simulink model "fourteen_bus_partial_linear"  (R2020b)
settings: Solver=VariableStepAuto  StartTime=0.0  StopTime=1  RelTol=1e-3
libraries: powerlib x95, powerlib_meascontrol x2
(part 1 of 2)
settings Model: Creator=aayushyaagarwal  LastModifiedBy=aayushyaagarwal

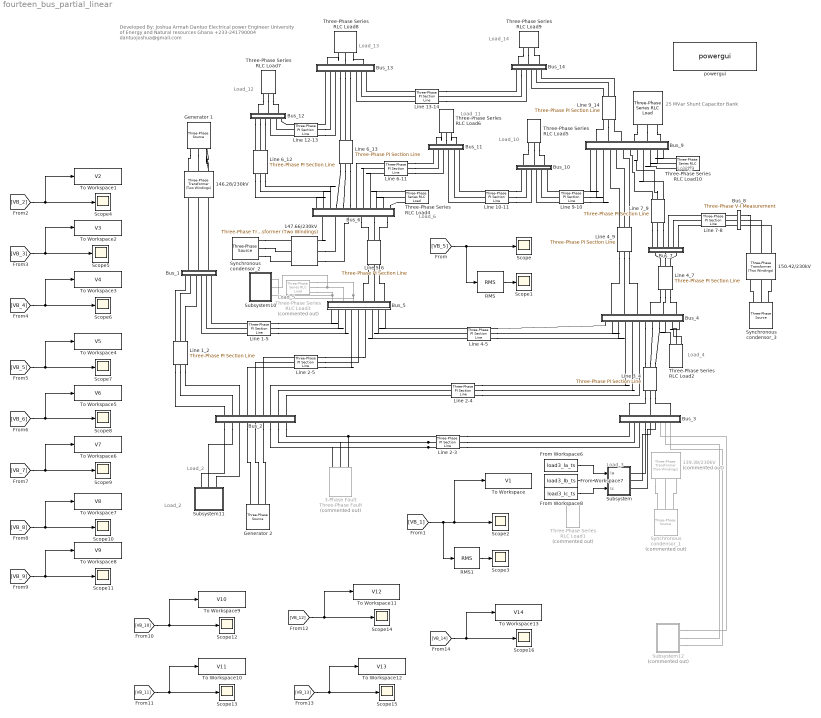
== system fourteen_bus_partial_linear ==
  note: Load_3
  note: Load_10
  note: Developed By:
      | Joshua Armah Dantuo
      | Electrical power Engineer
      | University of Energy and Natural resources
      | Ghana
      | +233-241790004
      | dantuojoshua@gmail.com
  note: Load_5
  note: Load_11
  note: Load_4
  note: Load_14
  note: Load_2
  note: Load_6
  note: Load_9
  note: Load_12
  note: Load_13
  note: 25 MVar Shunt
      | Capacitor Bank
  note: Load_2
  " " : powerlib/Elements/Three-Phase Series RLC Load  LConnTagsString=A|B|C  Configuration=Y (grounded)  NominalVoltage=230e3  Vabc=[1e3 1e3 1e3]  Vabcp=[1e3 1e3 1e3]  NominalFrequency=60  UnbalancedPower=off  ActivePower=0  InductivePower=0  CapacitivePower=25e6  Pabc=[10e3 9e3 11e3]  QLabc=[100 90 110]  QCabc=[100 90 110]  Pabcp=[10e3 9e3 11e3]  QLabcp=[100 90 110]  QCabcp=[100 90 110]  Measurements=None  LoadType=constant Z
  139.38/230kV : powerlib/Elements/Three-Phase Transformer (Two Windings)  Commented=on  Winding1Connection=Yg  Winding2Connection=Yg  CoreType=Three single-phase transformers  SetSaturation=off  Hysteresis=off  DataFile='hysteresis'  SetInitialFlux=off  Measurements=None  UNITS=pu  NominalPower=[ 120e6 , 60 ]  Winding1=[139.38e3 , 0.002 , 0.08 ]  Winding2=[ 230e3 , 0.002 , 0.08 ]  Rm=500  Lm=500  L0=0.5  Saturation=[ 0,0 ; 0.0024,1.2 ; 1.0,1.52 ]  InitialFluxes=[ 0.8 , -0.8 , 0.7 ]  BreakLoop=off  DiscreteSolver=Trapezoidal iterative  DataType=off  TransfoNumber=1
  146.28/230kV : powerlib/Elements/Three-Phase Transformer (Two Windings)  Winding1Connection=Yg  Winding2Connection=Yg  CoreType=Three single-phase transformers  SetSaturation=off  Hysteresis=off  DataFile='hysteresis'  SetInitialFlux=off  Measurements=None  UNITS=pu  NominalPower=[ 120e6 , 60 ]  Winding1=[146.28e3 , 0.002 , 0.08 ]  Winding2=[ 230e3 , 0.002 , 0.08 ]  Rm=500  Lm=500  L0=0.5  Saturation=[ 0,0 ; 0.0024,1.2 ; 1.0,1.52 ]  InitialFluxes=[ 0.8 , -0.8 , 0.7 ]  BreakLoop=off  DiscreteSolver=Trapezoidal iterative  DataType=off  TransfoNumber=1
  147.66/230kV : powerlib/Elements/Three-Phase Transformer (Two Windings)  Winding1Connection=Yg  Winding2Connection=Yg  CoreType=Three single-phase transformers  SetSaturation=off  Hysteresis=off  DataFile='hysteresis'  SetInitialFlux=off  Measurements=None  UNITS=pu  NominalPower=[ 120e6 , 60 ]  Winding1=[147.66e3 , 0.002 , 0.08 ]  Winding2=[ 230e3 , 0.002 , 0.08 ]  Rm=500  Lm=500  L0=0.5  Saturation=[ 0,0 ; 0.0024,1.2 ; 1.0,1.52 ]  InitialFluxes=[ 0.8 , -0.8 , 0.7 ]  BreakLoop=off  DiscreteSolver=Trapezoidal iterative  DataType=off  TransfoNumber=1
  150.42/230kV : powerlib/Elements/Three-Phase Transformer (Two Windings)  Winding1Connection=Yg  Winding2Connection=Yg  CoreType=Three single-phase transformers  SetSaturation=off  Hysteresis=off  DataFile='hysteresis'  SetInitialFlux=off  Measurements=None  UNITS=pu  NominalPower=[ 120e6 , 60 ]  Winding1=[150.42e3 , 0.002 , 0.08 ]  Winding2=[ 230e3 , 0.002 , 0.08 ]  Rm=500  Lm=500  L0=0.5  Saturation=[ 0,0 ; 0.0024,1.2 ; 1.0,1.52 ]  InitialFluxes=[ 0.8 , -0.8 , 0.7 ]  BreakLoop=off  DiscreteSolver=Trapezoidal iterative  DataType=off  TransfoNumber=1
  3-Phase Fault : powerlib/Elements/Three-Phase Fault  Commented=on  InitialStates=0  FaultA=on  FaultB=on  FaultC=on  GroundFault=on  SwitchTimes=[ 1 2]  External=off  SwitchStatus=NaN  FaultResistance=1e-3  GroundResistance=1e-3  SnubberResistance=inf  SnubberCapacitance=inf  Measurements=None
  Bus_1 : Subsystem
  Bus_10 : Subsystem
  Bus_11 : Subsystem
  Bus_12 : Subsystem
  Bus_13 : Subsystem
  Bus_14 : Subsystem
  Bus_2 : Subsystem
  Bus_3 : Subsystem
  Bus_4 : Subsystem
  Bus_5 : Subsystem
  Bus_6 : Subsystem
  Bus_7 : Subsystem
  Bus_8 : powerlib/Measurements/Three-Phase V-I Measurement  VoltageMeasurement=phase-to-phase  SetLabelV=on  LabelV=VB_8  Vpu=off  VpuLL=off  CurrentMeasurement=yes  SetLabelI=on  LabelI=IB_8  Ipu=off  Pbase=100e6  Vbase=500e3  OutputType=Complex  PhasorSimulation=off  PSBequivalent=0
  Bus_9 : Subsystem
  From Workspace6 : FromWorkspace  VariableName=load3_Ia_ts
  From Workspace7 : FromWorkspace  VariableName=load3_Ib_ts
  From Workspace8 : FromWorkspace  VariableName=load3_Ic_ts
  Generator 1 : powerlib/Electrical Sources/Three-Phase Source  InternalConnection=Yg  VoltagePhases=off  Voltage=(146280)*1.03071  PhaseAngle=3.7708  Voltage_phases=[25e3 25e3 25e3]/sqrt(3)  PhaseAngles_phases=[0 -120 +120]  Frequency=60  NonIdealSource=on  SpecifyImpedance=off  Resistance=0.8929  Inductance=16.58e-3  ShortCircuitLevel=100e6  BaseVoltage=146.28e3  XRratio=7  BusType=PV  Pref=163e6  Qref=0  Prefabc=[10e3, 10e3, 10e3]  Qrefabc=[0, 0, 0]  Qmin=-inf  Qmax=inf
  Generator 2 : powerlib/Electrical Sources/Three-Phase Source  InternalConnection=Yg  VoltagePhases=off  Voltage=(144210)*1.01655  PhaseAngle=-15.8323  Voltage_phases=[25e3 25e3 25e3]/sqrt(3)  PhaseAngles_phases=[0 -120 +120]  Frequency=60  NonIdealSource=on  SpecifyImpedance=off  Resistance=0.8929  Inductance=16.58e-3  ShortCircuitLevel=100e6  BaseVoltage=144.21e3  XRratio=7  BusType=PV  Pref=90e6  Qref=0  Prefabc=[10e3, 10e3, 10e3]  Qrefabc=[0, 0, 0]  Qmin=-inf  Qmax=inf
  Line 1-5 : powerlib/Elements/Three-Phase PI Section Line  LConnTagsString=a|b|c  RConnTagsString=A|B|C  Length=78.64  Frequency=60  Resistances=[ 0.3029 0.9086]  Inductances=[ 0.0033 0.0099]  Capacitances=[3.35e-7 1.01e-7]
  Line 10-11 : powerlib/Elements/Three-Phase PI Section Line  LConnTagsString=a|b|c  RConnTagsString=A|B|C  Length=4.93  Frequency=60  Resistances=[ 0.3667 1.1002]  Inductances=[ 0.0023 0.0068]  Capacitances=[1.22e-8 3.66e-8]
  Line 12-13 : powerlib/Elements/Three-Phase PI Section Line  LConnTagsString=a|b|c  RConnTagsString=A|B|C  Length=5.03  Frequency=60  Resistances=[ 0.9679 2.9038]  Inductances=[ 0.0023 0.0070]  Capacitances=[1.20e-8 3.59e-8]
  Line 13-14 : powerlib/Elements/Three-Phase PI Section Line  LConnTagsString=a|b|c  RConnTagsString=A|B|C  Length=6.64  Frequency=60  Resistances=[ 0.5676 1.7027]  Inductances=[ 0.0031 0.0092]  Capacitances=[9.06e-9 2.72e-9]
  Line 1_2 : powerlib/Elements/Three-Phase PI Section Line  LConnTagsString=a|b|c  RConnTagsString=A|B|C  Length=44.47  Frequency=60  Resistances=[ 0.1921 0.5763]  Inductances=[ 0.0016 0.0047]  Capacitances=[7.14e-9 2.14e-8]
  Line 2-3 : powerlib/Elements/Three-Phase PI Section Line  LConnTagsString=a|b|c  RConnTagsString=A|B|C  Length=68.47  Frequency=60  Resistances=[ 0.3026 0.9077]  Inductances=[ 0.0034 0.0101]  Capacitances=[3.29e-9 9.86e-8]
  Line 2-4 : powerlib/Elements/Three-Phase PI Section Line  LConnTagsString=a|b|c  RConnTagsString=A|B|C  Length=74.11  Frequency=60  Resistances=[ 0.3457 1.0370]  Inductances=[ 0.0028 0.0083]  Capacitances=[3.99e-9 1.20e-8]
  Line 2-5 : powerlib/Elements/Three-Phase PI Section Line  LConnTagsString=a|b|c  RConnTagsString=A|B|C  Length=61.18  Frequency=60  Resistances=[ 0.4104 1.2311]  Inductances=[ 0.0033 0.0100]  Capacitances=[3.34e-8 1.0e-8]
  Line 3_4 : powerlib/Elements/Three-Phase PI Section Line  LConnTagsString=a|b|c  RConnTagsString=A|B|C  Length=61.21  Frequency=60  Resistances=[ 0.4826 1.4479]  Inductances=[ 0.0033 0.0098]  Capacitances=[3.4e-9 1.02e-8]
  Line 4-5 : powerlib/Elements/Three-Phase PI Section Line  LConnTagsString=a|b|c  RConnTagsString=A|B|C  Length=18.47  Frequency=60  Resistances=[ 0.3186 0.9558]  Inductances=[ 0.0027 0.0080]  Capacitances=[4.17e-9 1.25e-8]
  Line 4_7 : powerlib/Elements/Three-Phase PI Section Line  LConnTagsString=a|b|c  RConnTagsString=A|B|C  Length=5.15  Frequency=60  Resistances=[ 0.0001 0.0003]  Inductances=[ 0.0475 0.1425]  Capacitances=[2.34e-10 7.02e-10]
  Line 4_9 : powerlib/Elements/Three-Phase PI Section Line  LConnTagsString=a|b|c  RConnTagsString=A|B|C  Length=8.39  Frequency=60  Resistances=[ 0.0001 0.0003]  Inductances=[ 0.0775 0.2325]  Capacitances=[1.43e-8 4.3e-8]
  Line 5_6 : powerlib/Elements/Three-Phase PI Section Line  LConnTagsString=a|b|c  RConnTagsString=A|B|C  Length=5.65  Frequency=60  Resistances=[ 0.0001 0.0003]  Inductances=[ 0.0522 0.1565]  Capacitances=[2.13e-10 6.39e-10]
  Line 6-11 : powerlib/Elements/Three-Phase PI Section Line  LConnTagsString=a|b|c  RConnTagsString=A|B|C  Length=5.02  Frequency=60  Resistances=[ 0.4172 1.2515]  Inductances=[ 0.0023 0.0070]  Capacitances=[1.20e-8 3.60e-8]
  Line 6_12 : powerlib/Elements/Three-Phase PI Section Line  LConnTagsString=a|b|c  RConnTagsString=A|B|C  Length=5.69  Frequency=60  Resistances=[ 0.4760 1.4281]  Inductances=[ 0.0026 0.0079]  Capacitances=[1.06e-8 3.17e-8]
  Line 6_13 : powerlib/Elements/Three-Phase PI Section Line  LConnTagsString=a|b|c  RConnTagsString=A|B|C  Length=4.06  Frequency=60  Resistances=[ 0.3590 1.0770]  Inductances=[ 0.0019 0.0056]  Capacitances=[1.48e-8 4.44e-8]
  Line 7-8 : powerlib/Elements/Three-Phase PI Section Line  LConnTagsString=a|b|c  RConnTagsString=A|B|C  Length=4.72  Frequency=60  Resistances=[ 0.0005 0.0014]  Inductances=[ 0.0022 0.0065]  Capacitances=[ 1.27e-8 3.82e-8]
  Line 7_9 : powerlib/Elements/Three-Phase PI Section Line  LConnTagsString=a|b|c  RConnTagsString=A|B|C  Length=3.73  Frequency=60  Resistances=[ 0.0006 0.0018]  Inductances=[ 0.0017 0.0052]  Capacitances=[ 1.61e-8 4.84e-8]
  Line 9-10 : powerlib/Elements/Three-Phase PI Section Line  LConnTagsString=a|b|c  RConnTagsString=A|B|C  Length=3.27  Frequency=60  Resistances=[ 0.2144 0.6431]  Inductances=[ 0.015 0.045]  Capacitances=[1.84e-9 5.52e-9]
  Line 9_14 : powerlib/Elements/Three-Phase PI Section Line  LConnTagsString=a|b|c  RConnTagsString=A|B|C  Length=69.85  Frequency=60  Resistances=[ 0.4788 1.4365]  Inductances=[ 0.027 0.081]  Capacitances=[1.03e-9 3.08e-9]
  RMS : powerlib_meascontrol/Measurements/RMS  TrueRMS=on  Freq=60  RMSInit=120  Ts=0
  RMS1 : powerlib_meascontrol/Measurements/RMS  TrueRMS=on  Freq=60  RMSInit=120  Ts=0
  Scope{,1..16} (17 alike) : Scope
  Subsystem : Subsystem
  Subsystem10 : Subsystem
  Subsystem11 : Subsystem
  Subsystem12 : Subsystem  Commented=on
  Synchronous condensor_1 : powerlib/Electrical Sources/Three-Phase Source  Commented=on  InternalConnection=Yg  VoltagePhases=off  Voltage=(139380)*1.01137  PhaseAngle=-34.48  Voltage_phases=[25e3 25e3 25e3]/sqrt(3)  PhaseAngles_phases=[0 -120 +120]  Frequency=60  NonIdealSource=on  SpecifyImpedance=off  Resistance=0.8929  Inductance=16.58e-3  ShortCircuitLevel=100e6  BaseVoltage=139.38e3  XRratio=7  BusType=PV  Pref=0  Qref=50.096e6  Prefabc=[10e3, 10e3, 10e3]  Qrefabc=[0, 0, 0]  Qmin=-inf  Qmax=inf
  Synchronous condensor_2 : powerlib/Electrical Sources/Three-Phase Source  InternalConnection=Yg  VoltagePhases=off  Voltage=(147660)*0.984306  PhaseAngle=-36.2022  Voltage_phases=[25e3 25e3 25e3]/sqrt(3)  PhaseAngles_phases=[0 -120 +120]  Frequency=60  NonIdealSource=on  SpecifyImpedance=off  Resistance=0.8929  Inductance=16.58e-3  ShortCircuitLevel=100e6  BaseVoltage=147.66e3  XRratio=7  BusType=PQ  Pref=0  Qref=25.276e6  Prefabc=[10e3, 10e3, 10e3]  Qrefabc=[0, 0, 0]  Qmin=-inf  Qmax=inf
  Synchronous condensor_3 : powerlib/Electrical Sources/Three-Phase Source  InternalConnection=Yg  VoltagePhases=off  Voltage=(150420)*0.995122  PhaseAngle=-36.1424  Voltage_phases=[25e3 25e3 25e3]/sqrt(3)  PhaseAngles_phases=[0 -120 +120]  Frequency=60  NonIdealSource=on  SpecifyImpedance=off  Resistance=0.8929  Inductance=16.58e-3  ShortCircuitLevel=100e6  BaseVoltage=150.42e3  XRratio=7  BusType=PQ  Pref=0  Qref=30.144e6  Prefabc=[10e3, 10e3, 10e3]  Qrefabc=[0, 0, 0]  Qmin=-inf  Qmax=inf
  Three-Phase Series RLC Load1 : powerlib/Elements/Three-Phase Series RLC Load  Commented=on  LConnTagsString=A|B|C  Configuration=Y (grounded)  NominalVoltage=(230000)*0.92821  Vabc=[1e3 1e3 1e3]  Vabcp=[1e3 1e3 1e3]  NominalFrequency=60  UnbalancedPower=off  ActivePower=113.04e6  InductivePower=22.8e6  CapacitivePower=0  Pabc=[10e3 9e3 11e3]  QLabc=[100 90 110]  QCabc=[100 90 110]  Pabcp=[10e3 9e3 11e3]  QLabcp=[100 90 110]  QCabcp=[100 90 110]  Measurements=None  LoadType=constant PQ
  Three-Phase Series RLC Load10 : powerlib/Elements/Three-Phase Series RLC Load  LConnTagsString=A|B|C  Configuration=Y (grounded)  NominalVoltage=(230000)*0.942986  Vabc=[1e3 1e3 1e3]  Vabcp=[1e3 1e3 1e3]  NominalFrequency=60  UnbalancedPower=off  ActivePower=35.4e6  InductivePower=19.92e6  CapacitivePower=0  Pabc=[10e3 9e3 11e3]  QLabc=[100 90 110]  QCabc=[100 90 110]  Pabcp=[10e3 9e3 11e3]  QLabcp=[100 90 110]  QCabcp=[100 90 110]  Measurements=None  LoadType=constant PQ
  Three-Phase Series RLC Load2 : powerlib/Elements/Three-Phase Series RLC Load  LConnTagsString=A|B|C  Configuration=Y (grounded)  NominalVoltage=(230000)*0.927953  Vabc=[1e3 1e3 1e3]  Vabcp=[1e3 1e3 1e3]  NominalFrequency=60  UnbalancedPower=off  ActivePower=57.36e6  InductivePower=0  CapacitivePower=4.68e6  Pabc=[10e3 9e3 11e3]  QLabc=[100 90 110]  QCabc=[100 90 110]  Pabcp=[10e3 9e3 11e3]  QLabcp=[100 90 110]  QCabcp=[100 90 110]  Measurements=None  LoadType=constant PQ
  Three-Phase Series RLC Load3 : powerlib/Elements/Three-Phase Series RLC Load  Commented=on  LConnTagsString=A|B|C  Configuration=Y (grounded)  NominalVoltage=(230000)*0.931217  Vabc=[1e3 1e3 1e3]  Vabcp=[1e3 1e3 1e3]  NominalFrequency=60  UnbalancedPower=off  ActivePower=9.12e6  InductivePower=1.92e6  CapacitivePower=0  Pabc=[10e3 9e3 11e3]  QLabc=[100 90 110]  QCabc=[100 90 110]  Pabcp=[10e3 9e3 11e3]  QLabcp=[100 90 110]  QCabcp=[100 90 110]  Measurements=None  LoadType=constant PQ
  Three-Phase Series RLC Load4 : powerlib/Elements/Three-Phase Series RLC Load  LConnTagsString=A|B|C  Configuration=Y (grounded)  NominalVoltage=(230000)*0.942548  Vabc=[1e3 1e3 1e3]  Vabcp=[1e3 1e3 1e3]  NominalFrequency=60  UnbalancedPower=off  ActivePower=13.44e6  InductivePower=9e6  CapacitivePower=0  Pabc=[10e3 9e3 11e3]  QLabc=[100 90 110]  QCabc=[100 90 110]  Pabcp=[10e3 9e3 11e3]  QLabcp=[100 90 110]  QCabcp=[100 90 110]  Measurements=None  LoadType=constant PQ
  Three-Phase Series RLC Load5 : powerlib/Elements/Three-Phase Series RLC Load  LConnTagsString=A|B|C  Configuration=Y (grounded)  NominalVoltage=(230000)*0.942502  Vabc=[1e3 1e3 1e3]  Vabcp=[1e3 1e3 1e3]  NominalFrequency=60  UnbalancedPower=off  ActivePower=10.8e6  InductivePower=6.96e6  CapacitivePower=0  Pabc=[10e3 9e3 11e3]  QLabc=[100 90 110]  QCabc=[100 90 110]  Pabcp=[10e3 9e3 11e3]  QLabcp=[100 90 110]  QCabcp=[100 90 110]  Measurements=None  LoadType=constant PQ
  Three-Phase Series RLC Load6 : powerlib/Elements/Three-Phase Series RLC Load  LConnTagsString=A|B|C  Configuration=Y (grounded)  NominalVoltage=(230000)*0.942338  Vabc=[1e3 1e3 1e3]  Vabcp=[1e3 1e3 1e3]  NominalFrequency=60  UnbalancedPower=off  ActivePower=4.2e6  InductivePower=2.16e6  CapacitivePower=0  Pabc=[10e3 9e3 11e3]  QLabc=[100 90 110]  QCabc=[100 90 110]  Pabcp=[10e3 9e3 11e3]  QLabcp=[100 90 110]  QCabcp=[100 90 110]  Measurements=None  LoadType=constant PQ
  Three-Phase Series RLC Load7 : powerlib/Elements/Three-Phase Series RLC Load  LConnTagsString=A|B|C  Configuration=Y (grounded)  NominalVoltage=(230000)*0.941818  Vabc=[1e3 1e3 1e3]  Vabcp=[1e3 1e3 1e3]  NominalFrequency=60  UnbalancedPower=off  ActivePower=7.32e6  InductivePower=1.92e6  CapacitivePower=0  Pabc=[10e3 9e3 11e3]  QLabc=[100 90 110]  QCabc=[100 90 110]  Pabcp=[10e3 9e3 11e3]  QLabcp=[100 90 110]  QCabcp=[100 90 110]  Measurements=None  LoadType=constant PQ
  Three-Phase Series RLC Load8 : powerlib/Elements/Three-Phase Series RLC Load  LConnTagsString=A|B|C  Configuration=Y (grounded)  NominalVoltage=(230000)*0.941642  Vabc=[1e3 1e3 1e3]  Vabcp=[1e3 1e3 1e3]  NominalFrequency=60  UnbalancedPower=off  ActivePower=16.2e6  InductivePower=6.96e6  CapacitivePower=0  Pabc=[10e3 9e3 11e3]  QLabc=[100 90 110]  QCabc=[100 90 110]  Pabcp=[10e3 9e3 11e3]  QLabcp=[100 90 110]  QCabcp=[100 90 110]  Measurements=None  LoadType=constant PQ
  Three-Phase Series RLC Load9 : powerlib/Elements/Three-Phase Series RLC Load  LConnTagsString=A|B|C  Configuration=Y (grounded)  NominalVoltage=(230000)*0.941422  Vabc=[1e3 1e3 1e3]  Vabcp=[1e3 1e3 1e3]  NominalFrequency=60  UnbalancedPower=off  ActivePower=17.88e6  InductivePower=6e6  CapacitivePower=0  Pabc=[10e3 9e3 11e3]  QLabc=[100 90 110]  QCabc=[100 90 110]  Pabcp=[10e3 9e3 11e3]  QLabcp=[100 90 110]  QCabcp=[100 90 110]  Measurements=None  LoadType=constant PQ
  To Workspace : ToWorkspace  VariableName=V1  SaveFormat=Timeseries  SampleTime=-1
  To Workspace1 : ToWorkspace  VariableName=V2  SaveFormat=Timeseries  SampleTime=-1
  To Workspace10 : ToWorkspace  VariableName=V11  SaveFormat=Timeseries  SampleTime=-1
  To Workspace11 : ToWorkspace  VariableName=V12  SaveFormat=Timeseries  SampleTime=-1
  To Workspace12 : ToWorkspace  VariableName=V13  SaveFormat=Timeseries  SampleTime=-1
  To Workspace13 : ToWorkspace  VariableName=V14  SaveFormat=Timeseries  SampleTime=-1
  To Workspace2 : ToWorkspace  VariableName=V3  SaveFormat=Timeseries  SampleTime=-1
  To Workspace3 : ToWorkspace  VariableName=V4  SaveFormat=Timeseries  SampleTime=-1
  To Workspace4 : ToWorkspace  VariableName=V5  SaveFormat=Timeseries  SampleTime=-1
  To Workspace5 : ToWorkspace  VariableName=V6  SaveFormat=Timeseries  SampleTime=-1
  To Workspace6 : ToWorkspace  VariableName=V7  SaveFormat=Timeseries  SampleTime=-1
  To Workspace7 : ToWorkspace  VariableName=V8  SaveFormat=Timeseries  SampleTime=-1
  To Workspace8 : ToWorkspace  VariableName=V9  SaveFormat=Timeseries  SampleTime=-1
  To Workspace9 : ToWorkspace  VariableName=V10  SaveFormat=Timeseries  SampleTime=-1
  powergui : powerlib/powergui  Priority=1  SimulationMode=Discrete  SampleTime=50e-6  frequency=60  Iterations=50  frequencyindice=60  Pbase=120e6  ErrMax=0.0001  UnitsV=kV  UnitsW=MW  buscounter=0  FunctionMessages=off  echomessages=off  EnableUseOfTLC=off  CurrentSourceSwitches=off  DisableSnubberDevices=off  DisableRonSwitches=off  DisableVfSwitches=off  DisplayEquations=off  AutomaticDiscreteSolvers=off  SolverType=Tustin/Backward Euler (TBE)  Interpol=off  ExternalGateDelay=off  methode=off  Ts=100  x0status=steady  SPID=on  SwTol=0  HookPort=off  NonlinearTolerance=1e-4  nMaxIteration=100  ContinueOnMaxIteration=off  RestoreLinks=warning  ResistiveCurrentMeasurement=off  Frange=[0:2:500]  Ylog=off  Xlog=on  ShowGrid=off  save=off  variable=ZData  structure=0  ZoomFFT=off  StartTime=0.0  cycles=1  DisplayStyle=1  fundamental=60  FreqAxis=off  MaxFrequency=1000  frequencyindicesteady=1  RmsSteady=1  display=off
  wires:
  [VB_4] -> To Workspace3/1, Scope6/1
  [VB_8] -> To Workspace7/1, Scope10/1
  RMS1/1 -> Scope3/1
  [VB_2] -> To Workspace1/1, Scope4/1
  [VB_7] -> To Workspace6/1, Scope9/1
  [VB_12] -> To Workspace11/1, Scope14/1
  [VB_13] -> To Workspace12/1, Scope15/1
  RMS/1 -> Scope1/1
  [VB_10] -> To Workspace9/1, Scope12/1
  [VB_5] -> RMS/1, Scope/1
  [VB_6] -> To Workspace5/1, Scope8/1
  [VB_14] -> To Workspace13/1, Scope16/1
  [VB_11] -> To Workspace10/1, Scope13/1
  [VB_1] -> RMS1/1, To Workspace/1, Scope2/1
  [VB_5] -> To Workspace4/1, Scope7/1
  [VB_3] -> To Workspace2/1, Scope5/1
  [VB_9] -> To Workspace8/1, Scope11/1
  From Workspace6/1 -> Subsystem/1(Ia)
  From Workspace7/1 -> Subsystem/2(Ib)
  From Workspace8/1 -> Subsystem/3(Ic)
  connections:
  Bus_2/RConn9 -- 3-Phase Fault/LConn3 -- Line 2-3/LConn1
  Line 2-3/LConn3 -- Bus_2/RConn7 -- 3-Phase Fault/LConn1
  Line 2-3/LConn2 -- Bus_2/RConn8 -- 3-Phase Fault/LConn2
  Line 7_9/RConn1 -- Bus_7/RConn1
  Bus_2/RConn6 -- Generator 2/RConn3
  Line 5_6/RConn1 -- Bus_5/LConn4
  Bus_8/LConn1 -- Line 7-8/RConn1
  Line 12-13/LConn1 -- Bus_12/RConn6
  Three-Phase Series RLC Load4/LConn2 -- Bus_6/RConn11
  Line 6-11/RConn3 -- Bus_11/RConn3
  Line 6-11/RConn2 -- Bus_11/RConn2
  Line 1_2/RConn1 -- Bus_2/LConn1
  Line 6_12/RConn3 -- Bus_6/RConn3
  Line 5_6/RConn2 -- Bus_5/LConn5
  Line 10-11/LConn1 -- Bus_11/RConn6
  Line 1-5/RConn3 -- Bus_5/RConn3
  Line 10-11/RConn3 -- Bus_10/RConn3
  Three-Phase Series RLC Load8/LConn1 -- Bus_13/LConn1
  Line 12-13/LConn2 -- Bus_12/RConn5
  Line 2-4/RConn3 -- Bus_4/RConn6
  Line 2-4/LConn2 -- Bus_2/LConn8
  Three-Phase Series RLC Load10/LConn2 -- Bus_9/RConn11
  Synchronous condensor_3/RConn3 -- 150.42/230kV/LConn3
  Bus_2/RConn4 -- Generator 2/RConn1
  Three-Phase Series RLC Load3/LConn3 -- Subsystem10/RConn3 -- Bus_5/LConn1
  Synchronous condensor_2/RConn3 -- 147.66/230kV/LConn3
  Three-Phase Series RLC Load7/LConn2 -- Bus_12/LConn2
  Line 2-3/RConn1 -- Bus_3/RConn1
  Line 6_13/RConn3 -- Bus_6/RConn6
  " "/LConn2 -- Bus_9/LConn5
  Line 13-14/LConn3 -- Bus_13/RConn7
  Synchronous condensor_1/RConn3 -- 139.38/230kV/LConn3
  Bus_9/LConn3 -- Line 9_14/RConn3
  Three-Phase Series RLC Load9/LConn2 -- Bus_14/LConn2
  Bus_12/RConn3 -- Line 6_12/LConn3
  Line 4-5/RConn2 -- Bus_4/RConn2
  Line 4_9/LConn1 -- Bus_9/RConn4
  Line 4-5/RConn1 -- Bus_4/RConn1
  Line 6_12/RConn2 -- Bus_6/RConn2
  Line 2-5/LConn3 -- Bus_2/LConn4
  Line 4_7/RConn2 -- Bus_4/LConn5
  147.66/230kV/RConn2 -- Bus_6/LConn2
  139.38/230kV/LConn1 -- Synchronous condensor_1/RConn1
  Line 6_13/RConn2 -- Bus_6/RConn5
  Line 9-10/RConn1 -- Bus_9/RConn1
  Line 12-13/RConn1 -- Bus_13/RConn1
  Line 4_9/LConn2 -- Bus_9/RConn5
  Three-Phase Series RLC Load9/LConn1 -- Bus_14/LConn1
  Three-Phase Series RLC Load5/LConn1 -- Bus_10/LConn1
  Line 1-5/LConn2 -- Bus_1/RConn5
  Line 3_4/RConn2 -- Bus_3/LConn2
  Line 2-4/LConn1 -- Bus_2/LConn7
  Bus_6/LConn5 -- Line 5_6/LConn2
  Line 3_4/RConn3 -- Bus_3/LConn3
  Three-Phase Series RLC Load5/LConn3 -- Bus_10/LConn3
  Line 4_9/LConn3 -- Bus_9/RConn6
  Synchronous condensor_3/RConn1 -- 150.42/230kV/LConn1
  Three-Phase Series RLC Load3/LConn1 -- Subsystem10/RConn1 -- Bus_5/LConn3
  Three-Phase Series RLC Load8/LConn3 -- Bus_13/LConn3
  Line 2-3/RConn2 -- Bus_3/RConn2
  " "/LConn1 -- Bus_9/LConn4
  Line 9-10/RConn2 -- Bus_9/RConn2
  Bus_12/RConn1 -- Line 6_12/LConn1
  Line 6-11/RConn1 -- Bus_11/RConn1
  Line 12-13/LConn3 -- Bus_12/RConn4
  Three-Phase Series RLC Load4/LConn3 -- Bus_6/RConn12
  Line 1_2/RConn3 -- Bus_2/LConn3
  Line 1-5/LConn3 -- Bus_1/RConn4
  Line 2-5/RConn2 -- Bus_5/RConn5
  150.42/230kV/RConn2 -- Bus_8/RConn2
  Synchronous condensor_3/RConn2 -- 150.42/230kV/LConn2
  147.66/230kV/RConn3 -- Bus_6/LConn3
  Line 7_9/LConn1 -- Bus_9/RConn7
  Line 1-5/LConn1 -- Bus_1/RConn6
  Line 1_2/RConn2 -- Bus_2/LConn2
  Bus_14/RConn2 -- Line 13-14/RConn2
  Line 5_6/RConn3 -- Bus_5/LConn6
  Line 6_13/RConn1 -- Bus_6/RConn4
  Bus_13/RConn6 -- Line 6_13/LConn3
  Line 4_7/LConn1 -- Bus_7/LConn1
  Three-Phase Series RLC Load6/LConn1 -- Bus_11/LConn1
  Generator 1/RConn2 -- 146.28/230kV/LConn2
  Line 4-5/LConn3 -- Bus_5/RConn7
  Line 6-11/LConn1 -- Bus_6/RConn7
  Three-Phase Series RLC Load9/LConn3 -- Bus_14/LConn3
  Line 6_12/RConn1 -- Bus_6/RConn1
  Bus_4/RConn8 -- Line 3_4/LConn2
  Bus_8/LConn3 -- Line 7-8/RConn3
  Three-Phase Series RLC Load7/LConn3 -- Bus_12/LConn3
  Line 2-3/RConn3 -- Bus_3/RConn3
  Line 6-11/LConn2 -- Bus_6/RConn8
  Line 6-11/LConn3 -- Bus_6/RConn9
  Three-Phase Series RLC Load2/LConn2 -- Bus_4/RConn11
  Three-Phase Series RLC Load4/LConn1 -- Bus_6/RConn10
  Line 4-5/LConn1 -- Bus_5/RConn9
  Bus_6/LConn4 -- Line 5_6/LConn1
  Line 2-5/RConn3 -- Bus_5/RConn4
  Line 1-5/RConn1 -- Bus_5/RConn1
  Line 3_4/RConn1 -- Bus_3/LConn1
  Line 7-8/LConn3 -- Bus_7/RConn6
  Bus_8/RConn1 -- 150.42/230kV/RConn1
  Line 7_9/RConn2 -- Bus_7/RConn2
  Line 1-5/RConn2 -- Bus_5/RConn2
  Line 10-11/RConn1 -- Bus_10/RConn1
  Line 7-8/LConn1 -- Bus_7/RConn4
  Line 13-14/RConn3 -- Bus_14/RConn3
  Bus_4/RConn7 -- Line 3_4/LConn1
  Line 9_14/LConn1 -- Bus_14/RConn4
  Line 10-11/LConn2 -- Bus_11/RConn5
  Synchronous condensor_2/RConn1 -- 147.66/230kV/LConn1
  Line 4_9/RConn2 -- Bus_4/LConn2
  Line 9_14/RConn2 -- Bus_9/LConn2
  Line 2-4/RConn2 -- Bus_4/RConn5
  Line 9-10/LConn3 -- Bus_10/RConn4
  Line 9-10/LConn1 -- Bus_10/RConn6
  Synchronous condensor_1/RConn2 -- 139.38/230kV/LConn2
  Line 9-10/RConn3 -- Bus_9/RConn3
  Three-Phase Series RLC Load2/LConn3 -- Bus_4/RConn12
  Line 9-10/LConn2 -- Bus_10/RConn5
  Bus_12/RConn2 -- Line 6_12/LConn2
  Line 4-5/LConn2 -- Bus_5/RConn8
  Line 1_2/LConn3 -- Bus_1/RConn3
  Line 4_7/RConn1 -- Bus_4/LConn4
  Bus_2/LConn5 -- Line 2-5/LConn2
  Line 4-5/RConn3 -- Bus_4/RConn3
  " "/LConn3 -- Bus_9/LConn6
  Line 10-11/LConn3 -- Bus_11/RConn4
  Bus_13/RConn5 -- Line 6_13/LConn2
  Three-Phase Series RLC Load10/LConn1 -- Bus_9/RConn12
  Line 7_9/LConn3 -- Bus_9/RConn9
  Synchronous condensor_2/RConn2 -- 147.66/230kV/LConn2
  Line 13-14/LConn2 -- Bus_13/RConn8
  146.28/230kV/LConn1 -- Generator 1/RConn1
  Bus_4/RConn9 -- Line 3_4/LConn3
  Line 4_7/LConn3 -- Bus_7/LConn3
  Line 12-13/RConn3 -- Bus_13/RConn3
  Bus_8/LConn2 -- Line 7-8/RConn2
  Line 9_14/LConn2 -- Bus_14/RConn5
  Bus_9/LConn1 -- Line 9_14/RConn1
  Line 1_2/LConn1 -- Bus_1/RConn1
  Line 7-8/LConn2 -- Bus_7/RConn5
  Line 13-14/RConn1 -- Bus_14/RConn1
  Line 1_2/LConn2 -- Bus_1/RConn2
  Line 10-11/RConn2 -- Bus_10/RConn2
  150.42/230kV/RConn3 -- Bus_8/RConn3
  Line 4_7/RConn3 -- Bus_4/LConn6
  Line 4_9/RConn3 -- Bus_4/LConn3
  Three-Phase Series RLC Load7/LConn1 -- Bus_12/LConn1
  Three-Phase Series RLC Load10/LConn3 -- Bus_9/RConn10
  Line 7_9/RConn3 -- Bus_7/RConn3
  Bus_6/LConn6 -- Line 5_6/LConn3
  Bus_7/LConn2 -- Line 4_7/LConn2
  Line 2-5/RConn1 -- Bus_5/RConn6
  Three-Phase Series RLC Load6/LConn3 -- Bus_11/LConn3
  Line 2-5/LConn1 -- Bus_2/LConn6
  Line 4_9/RConn1 -- Bus_4/LConn1
  Line 9_14/LConn3 -- Bus_14/RConn6
  Three-Phase Series RLC Load5/LConn2 -- Bus_10/LConn2
  Line 7_9/LConn2 -- Bus_9/RConn8
  Line 2-4/LConn3 -- Bus_2/LConn9
  Three-Phase Series RLC Load3/LConn2 -- Subsystem10/RConn2 -- Bus_5/LConn2
  Line 13-14/LConn1 -- Bus_13/RConn9
  147.66/230kV/RConn1 -- Bus_6/LConn1
  Line 2-4/RConn1 -- Bus_4/RConn4
  Line 12-13/RConn2 -- Bus_13/RConn2
  Three-Phase Series RLC Load2/LConn1 -- Bus_4/RConn10
  Bus_2/RConn5 -- Generator 2/RConn2
  Generator 1/RConn3 -- 146.28/230kV/LConn3
  Three-Phase Series RLC Load8/LConn2 -- Bus_13/LConn2
  Three-Phase Series RLC Load6/LConn2 -- Bus_11/LConn2
  Bus_13/RConn4 -- Line 6_13/LConn1
  Bus_1/LConn2 -- 146.28/230kV/RConn2
  Bus_1/LConn3 -- 146.28/230kV/RConn1
  Bus_1/LConn1 -- 146.28/230kV/RConn3
  Bus_2/RConn2 -- Subsystem11/RConn2
  Bus_2/RConn1 -- Subsystem11/RConn1
  Subsystem11/RConn3 -- Bus_2/RConn3
  Bus_3/RConn4 -- Subsystem/RConn1
  Bus_3/RConn5 -- Subsystem/RConn2
  Bus_3/RConn6 -- Subsystem/RConn3
  Subsystem12/RConn1 -- Bus_3/RConn7
  Subsystem12/RConn2 -- Bus_3/RConn8
  Subsystem12/RConn3 -- Bus_3/RConn9

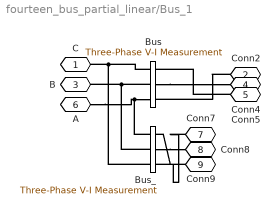
== system fourteen_bus_partial_linear/Bus_1 ==
  Bus : powerlib/Measurements/Three-Phase V-I Measurement  VoltageMeasurement=phase-to-phase  SetLabelV=on  LabelV=VB_1  Vpu=off  VpuLL=off  CurrentMeasurement=yes  SetLabelI=on  LabelI=IB_1  Ipu=off  Pbase=100e6  Vbase=500e3  OutputType=Complex  PhasorSimulation=off  PSBequivalent=0
  Bus_ : powerlib/Measurements/Three-Phase V-I Measurement  VoltageMeasurement=phase-to-phase  SetLabelV=on  LabelV=V_B1  Vpu=off  VpuLL=off  CurrentMeasurement=yes  SetLabelI=on  LabelI=I_B1  Ipu=off  Pbase=100e6  Vbase=500e3  OutputType=Complex  PhasorSimulation=off  PSBequivalent=0
  C : PMIOPort  Side=Left
  Conn2 : PMIOPort  Port=2  Side=Right
  B : PMIOPort  Port=3  Side=Left
  Conn4 : PMIOPort  Port=4  Side=Right
  Conn5 : PMIOPort  Port=5  Side=Right
  A : PMIOPort  Port=6  Side=Left
  Conn7 : PMIOPort  Port=7  Side=Right
  Conn8 : PMIOPort  Port=8  Side=Right
  Conn9 : PMIOPort  Port=9  Side=Right
  connections:
  A/RConn1 -- Bus_/LConn1 -- Bus/LConn3
  Bus/RConn2 -- Conn4/RConn1
  Bus_/RConn2 -- Conn8/RConn1
  Bus/LConn2 -- Bus_/LConn2 -- B/RConn1
  Bus/LConn1 -- Bus_/LConn3 -- C/RConn1
  Conn5/RConn1 -- Bus/RConn1
  Conn2/RConn1 -- Bus/RConn3
  Conn9/RConn1 -- Bus_/RConn1
  Conn7/RConn1 -- Bus_/RConn3

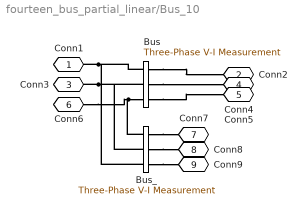
== system fourteen_bus_partial_linear/Bus_10 ==
  Bus : powerlib/Measurements/Three-Phase V-I Measurement  VoltageMeasurement=phase-to-phase  SetLabelV=on  LabelV=VB_10  Vpu=off  VpuLL=off  CurrentMeasurement=yes  SetLabelI=on  LabelI=IB_10  Ipu=off  Pbase=100e6  Vbase=500e3  OutputType=Complex  PhasorSimulation=off  PSBequivalent=0
  Bus_ : powerlib/Measurements/Three-Phase V-I Measurement  VoltageMeasurement=phase-to-phase  SetLabelV=on  LabelV=V_B10  Vpu=off  VpuLL=off  CurrentMeasurement=yes  SetLabelI=on  LabelI=I_B10  Ipu=off  Pbase=100e6  Vbase=500e3  OutputType=Complex  PhasorSimulation=off  PSBequivalent=0
  Conn1 : PMIOPort  Side=Left
  Conn2 : PMIOPort  Port=2  Side=Right
  Conn3 : PMIOPort  Port=3  Side=Left
  Conn4 : PMIOPort  Port=4  Side=Right
  Conn5 : PMIOPort  Port=5  Side=Right
  Conn6 : PMIOPort  Port=6  Side=Left
  Conn7 : PMIOPort  Port=7  Side=Right
  Conn8 : PMIOPort  Port=8  Side=Right
  Conn9 : PMIOPort  Port=9  Side=Right
  connections:
  Conn1/RConn1 -- Bus_/LConn3 -- Bus/LConn1
  Conn3/RConn1 -- Bus_/LConn2 -- Bus/LConn2
  Bus_/RConn2 -- Conn8/RConn1
  Bus/RConn2 -- Conn4/RConn1
  Bus/LConn3 -- Bus_/LConn1 -- Conn6/RConn1
  Bus_/RConn1 -- Conn7/RConn1
  Bus_/RConn3 -- Conn9/RConn1
  Bus/RConn1 -- Conn2/RConn1
  Bus/RConn3 -- Conn5/RConn1

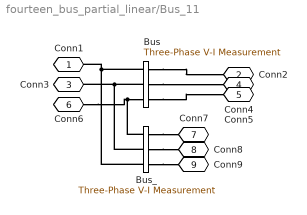
== system fourteen_bus_partial_linear/Bus_11 ==
  Bus : powerlib/Measurements/Three-Phase V-I Measurement  VoltageMeasurement=phase-to-phase  SetLabelV=on  LabelV=VB_11  Vpu=off  VpuLL=off  CurrentMeasurement=yes  SetLabelI=on  LabelI=IB_11  Ipu=off  Pbase=100e6  Vbase=500e3  OutputType=Complex  PhasorSimulation=off  PSBequivalent=0
  Bus_ : powerlib/Measurements/Three-Phase V-I Measurement  VoltageMeasurement=phase-to-phase  SetLabelV=on  LabelV=V_B11  Vpu=off  VpuLL=off  CurrentMeasurement=yes  SetLabelI=on  LabelI=I_B11  Ipu=off  Pbase=100e6  Vbase=500e3  OutputType=Complex  PhasorSimulation=off  PSBequivalent=0
  Conn1 : PMIOPort  Side=Left
  Conn2 : PMIOPort  Port=2  Side=Right
  Conn3 : PMIOPort  Port=3  Side=Left
  Conn4 : PMIOPort  Port=4  Side=Right
  Conn5 : PMIOPort  Port=5  Side=Right
  Conn6 : PMIOPort  Port=6  Side=Left
  Conn7 : PMIOPort  Port=7  Side=Right
  Conn8 : PMIOPort  Port=8  Side=Right
  Conn9 : PMIOPort  Port=9  Side=Right
  connections:
  Bus/RConn3 -- Conn5/RConn1
  Bus/RConn1 -- Conn2/RConn1
  Bus_/RConn3 -- Conn9/RConn1
  Bus_/RConn1 -- Conn7/RConn1
  Conn6/RConn1 -- Bus_/LConn1 -- Bus/LConn3
  Bus/RConn2 -- Conn4/RConn1
  Bus_/RConn2 -- Conn8/RConn1
  Bus/LConn2 -- Bus_/LConn2 -- Conn3/RConn1
  Bus/LConn1 -- Conn1/RConn1 -- Bus_/LConn3

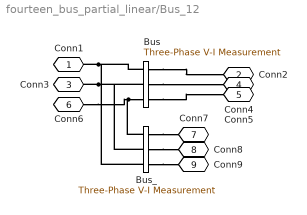
== system fourteen_bus_partial_linear/Bus_12 ==
  Bus : powerlib/Measurements/Three-Phase V-I Measurement  VoltageMeasurement=phase-to-phase  SetLabelV=on  LabelV=VB_12  Vpu=off  VpuLL=off  CurrentMeasurement=yes  SetLabelI=on  LabelI=IB_12  Ipu=off  Pbase=100e6  Vbase=500e3  OutputType=Complex  PhasorSimulation=off  PSBequivalent=0
  Bus_ : powerlib/Measurements/Three-Phase V-I Measurement  VoltageMeasurement=phase-to-phase  SetLabelV=on  LabelV=V_B12  Vpu=off  VpuLL=off  CurrentMeasurement=yes  SetLabelI=on  LabelI=I_B12  Ipu=off  Pbase=100e6  Vbase=500e3  OutputType=Complex  PhasorSimulation=off  PSBequivalent=0
  Conn1 : PMIOPort  Side=Left
  Conn2 : PMIOPort  Port=2  Side=Right
  Conn3 : PMIOPort  Port=3  Side=Left
  Conn4 : PMIOPort  Port=4  Side=Right
  Conn5 : PMIOPort  Port=5  Side=Right
  Conn6 : PMIOPort  Port=6  Side=Left
  Conn7 : PMIOPort  Port=7  Side=Right
  Conn8 : PMIOPort  Port=8  Side=Right
  Conn9 : PMIOPort  Port=9  Side=Right
  connections:
  Conn1/RConn1 -- Bus_/LConn3 -- Bus/LConn1
  Conn3/RConn1 -- Bus_/LConn2 -- Bus/LConn2
  Bus_/RConn2 -- Conn8/RConn1
  Bus/RConn2 -- Conn4/RConn1
  Bus/LConn3 -- Bus_/LConn1 -- Conn6/RConn1
  Bus_/RConn1 -- Conn7/RConn1
  Bus_/RConn3 -- Conn9/RConn1
  Bus/RConn1 -- Conn2/RConn1
  Bus/RConn3 -- Conn5/RConn1

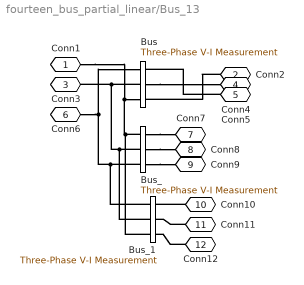
== system fourteen_bus_partial_linear/Bus_13 ==
  Bus : powerlib/Measurements/Three-Phase V-I Measurement  VoltageMeasurement=phase-to-phase  SetLabelV=on  LabelV=VB_13  Vpu=off  VpuLL=off  CurrentMeasurement=yes  SetLabelI=on  LabelI=IB_13  Ipu=off  Pbase=100e6  Vbase=500e3  OutputType=Complex  PhasorSimulation=off  PSBequivalent=0
  Bus_ : powerlib/Measurements/Three-Phase V-I Measurement  VoltageMeasurement=phase-to-phase  SetLabelV=on  LabelV=V_B13_13  Vpu=off  VpuLL=off  CurrentMeasurement=yes  SetLabelI=on  LabelI=I_B13_13  Ipu=off  Pbase=100e6  Vbase=500e3  OutputType=Complex  PhasorSimulation=off  PSBequivalent=0
  Bus_1 : powerlib/Measurements/Three-Phase V-I Measurement  VoltageMeasurement=phase-to-phase  SetLabelV=on  LabelV=V_B13  Vpu=off  VpuLL=off  CurrentMeasurement=yes  SetLabelI=on  LabelI=I_B13  Ipu=off  Pbase=100e6  Vbase=500e3  OutputType=Complex  PhasorSimulation=off  PSBequivalent=0
  Conn1 : PMIOPort  Side=Left
  Conn2 : PMIOPort  Port=2  Side=Right
  Conn3 : PMIOPort  Port=3  Side=Left
  Conn4 : PMIOPort  Port=4  Side=Right
  Conn5 : PMIOPort  Port=5  Side=Right
  Conn6 : PMIOPort  Port=6  Side=Left
  Conn7 : PMIOPort  Port=7  Side=Right
  Conn8 : PMIOPort  Port=8  Side=Right
  Conn9 : PMIOPort  Port=9  Side=Right
  Conn10 : PMIOPort  Port=10  Side=Right
  Conn11 : PMIOPort  Port=11  Side=Right
  Conn12 : PMIOPort  Port=12  Side=Right
  connections:
  Bus_1/LConn1 -- Bus_/LConn3 -- Conn6/RConn1 -- Bus/LConn1
  Conn3/RConn1 -- Bus/LConn2 -- Bus_1/LConn2 -- Bus_/LConn2
  Bus_/RConn2 -- Conn8/RConn1
  Bus/RConn2 -- Conn4/RConn1
  Bus_1/LConn3 -- Bus_/LConn1 -- Conn1/RConn1 -- Bus/LConn3
  Bus_/RConn1 -- Conn7/RConn1
  Bus_/RConn3 -- Conn9/RConn1
  Conn10/RConn1 -- Bus_1/RConn1
  Conn11/RConn1 -- Bus_1/RConn2
  Conn12/RConn1 -- Bus_1/RConn3
  Conn5/RConn1 -- Bus/RConn1
  Conn2/RConn1 -- Bus/RConn3

== system fourteen_bus_partial_linear/Bus_14 ==
  Bus : powerlib/Measurements/Three-Phase V-I Measurement  VoltageMeasurement=phase-to-phase  SetLabelV=on  LabelV=VB_14  Vpu=off  VpuLL=off  CurrentMeasurement=yes  SetLabelI=on  LabelI=IB_14  Ipu=off  Pbase=100e6  Vbase=500e3  OutputType=Complex  PhasorSimulation=off  PSBequivalent=0
  Bus_ : powerlib/Measurements/Three-Phase V-I Measurement  VoltageMeasurement=phase-to-phase  SetLabelV=on  LabelV=V_B14  Vpu=off  VpuLL=off  CurrentMeasurement=yes  SetLabelI=on  LabelI=I_B14  Ipu=off  Pbase=100e6  Vbase=500e3  OutputType=Complex  PhasorSimulation=off  PSBequivalent=0
  Conn1 : PMIOPort  Side=Left
  Conn2 : PMIOPort  Port=2  Side=Right
  Conn3 : PMIOPort  Port=3  Side=Left
  Conn4 : PMIOPort  Port=4  Side=Right
  Conn5 : PMIOPort  Port=5  Side=Right
  Conn6 : PMIOPort  Port=6  Side=Left
  Conn7 : PMIOPort  Port=7  Side=Right
  Conn8 : PMIOPort  Port=8  Side=Right
  Conn9 : PMIOPort  Port=9  Side=Right
  connections:
  Conn1/RConn1 -- Bus_/LConn3 -- Bus/LConn1
  Conn3/RConn1 -- Bus_/LConn2 -- Bus/LConn2
  Bus_/RConn2 -- Conn8/RConn1
  Bus/RConn2 -- Conn4/RConn1
  Bus/LConn3 -- Bus_/LConn1 -- Conn6/RConn1
  Bus/RConn1 -- Conn2/RConn1
  Bus/RConn3 -- Conn5/RConn1
  Conn7/RConn1 -- Bus_/RConn3
  Conn9/RConn1 -- Bus_/RConn1

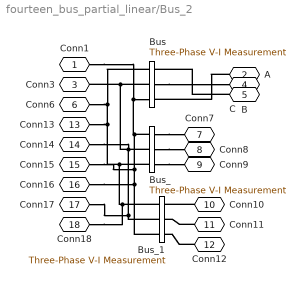
== system fourteen_bus_partial_linear/Bus_2 ==
  Bus : powerlib/Measurements/Three-Phase V-I Measurement  VoltageMeasurement=phase-to-phase  SetLabelV=on  LabelV=VB_2  Vpu=off  VpuLL=off  CurrentMeasurement=yes  SetLabelI=on  LabelI=IB_2  Ipu=off  Pbase=100e6  Vbase=500e3  OutputType=Complex  PhasorSimulation=off  PSBequivalent=0
  Bus_ : powerlib/Measurements/Three-Phase V-I Measurement  VoltageMeasurement=phase-to-phase  SetLabelV=on  LabelV=V_B22  Vpu=off  VpuLL=off  CurrentMeasurement=yes  SetLabelI=on  LabelI=I_B22  Ipu=off  Pbase=100e6  Vbase=500e3  OutputType=Complex  PhasorSimulation=off  PSBequivalent=0
  Bus_1 : powerlib/Measurements/Three-Phase V-I Measurement  VoltageMeasurement=phase-to-phase  SetLabelV=on  LabelV=V_B2  Vpu=off  VpuLL=off  CurrentMeasurement=yes  SetLabelI=on  LabelI=I_B2  Ipu=off  Pbase=100e6  Vbase=500e3  OutputType=Complex  PhasorSimulation=off  PSBequivalent=0
  Conn1 : PMIOPort  Side=Left
  A : PMIOPort  Port=2  Side=Right
  Conn3 : PMIOPort  Port=3  Side=Left
  B : PMIOPort  Port=4  Side=Right
  C : PMIOPort  Port=5  Side=Right
  Conn6 : PMIOPort  Port=6  Side=Left
  Conn7 : PMIOPort  Port=7  Side=Right
  Conn8 : PMIOPort  Port=8  Side=Right
  Conn9 : PMIOPort  Port=9  Side=Right
  Conn10 : PMIOPort  Port=10  Side=Right
  Conn11 : PMIOPort  Port=11  Side=Right
  Conn12 : PMIOPort  Port=12  Side=Right
  Conn13 : PMIOPort  Port=13  Side=Left
  Conn14 : PMIOPort  Port=14  Side=Left
  Conn15 : PMIOPort  Port=15  Side=Left
  Conn16 : PMIOPort  Port=16  Side=Left
  Conn17 : PMIOPort  Port=17  Side=Left
  Conn18 : PMIOPort  Port=18  Side=Left
  connections:
  Bus_1/LConn1 -- Conn18/RConn1 -- Bus_/LConn3 -- Conn13/RConn1 -- Bus/LConn1 -- Conn6/RConn1
  Conn3/RConn1 -- Bus/LConn2 -- Conn17/RConn1 -- Bus_1/LConn2 -- Conn14/RConn1 -- Bus_/LConn2
  Bus_/RConn2 -- Conn8/RConn1
  Bus/RConn2 -- B/RConn1
  Bus_1/LConn3 -- Conn16/RConn1 -- Conn15/RConn1 -- Bus_/LConn1 -- Conn1/RConn1 -- Bus/LConn3
  Bus_/RConn1 -- Conn7/RConn1
  Bus_/RConn3 -- Conn9/RConn1
  Conn10/RConn1 -- Bus_1/RConn1
  Conn11/RConn1 -- Bus_1/RConn2
  Conn12/RConn1 -- Bus_1/RConn3
  C/RConn1 -- Bus/RConn1
  A/RConn1 -- Bus/RConn3

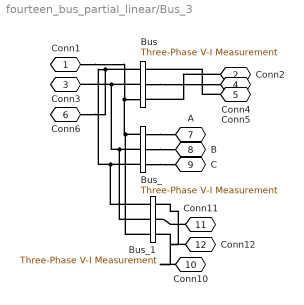
== system fourteen_bus_partial_linear/Bus_3 ==
  Bus : powerlib/Measurements/Three-Phase V-I Measurement  VoltageMeasurement=phase-to-phase  SetLabelV=on  LabelV=VB_3  Vpu=off  VpuLL=off  CurrentMeasurement=yes  SetLabelI=on  LabelI=IB_3  Ipu=off  Pbase=100e6  Vbase=500e3  OutputType=Complex  PhasorSimulation=off  PSBequivalent=0
  Bus_ : powerlib/Measurements/Three-Phase V-I Measurement  VoltageMeasurement=phase-to-phase  SetLabelV=on  LabelV=V_B33  Vpu=off  VpuLL=off  CurrentMeasurement=yes  SetLabelI=on  LabelI=I_B33  Ipu=off  Pbase=100e6  Vbase=500e3  OutputType=Complex  PhasorSimulation=off  PSBequivalent=0
  Bus_1 : powerlib/Measurements/Three-Phase V-I Measurement  VoltageMeasurement=phase-to-phase  SetLabelV=on  LabelV=V_B3  Vpu=off  VpuLL=off  CurrentMeasurement=yes  SetLabelI=on  LabelI=I_B3  Ipu=off  Pbase=100e6  Vbase=500e3  OutputType=Complex  PhasorSimulation=off  PSBequivalent=0
  Conn1 : PMIOPort  Side=Left
  Conn2 : PMIOPort  Port=2  Side=Right
  Conn3 : PMIOPort  Port=3  Side=Left
  Conn4 : PMIOPort  Port=4  Side=Right
  Conn5 : PMIOPort  Port=5  Side=Right
  Conn6 : PMIOPort  Port=6  Side=Left
  A : PMIOPort  Port=7  Side=Right
  B : PMIOPort  Port=8  Side=Right
  C : PMIOPort  Port=9  Side=Right
  Conn10 : PMIOPort  Port=10  Side=Right
  Conn11 : PMIOPort  Port=11  Side=Right
  Conn12 : PMIOPort  Port=12  Side=Right
  connections:
  Conn11/RConn1 -- Bus_1/RConn2
  Bus_/RConn3 -- C/RConn1
  Bus_/RConn1 -- A/RConn1
  Bus_1/LConn3 -- Bus_/LConn1 -- Conn1/RConn1 -- Bus/LConn3
  Bus/RConn2 -- Conn4/RConn1
  Bus_/RConn2 -- B/RConn1
  Bus_1/LConn2 -- Bus_/LConn2 -- Bus/LConn2 -- Conn3/RConn1
  Bus_/LConn3 -- Bus_1/LConn1 -- Conn6/RConn1 -- Bus/LConn1
  Conn10/RConn1 -- Bus_1/RConn3
  Conn12/RConn1 -- Bus_1/RConn1
  Conn2/RConn1 -- Bus/RConn3
  Conn5/RConn1 -- Bus/RConn1

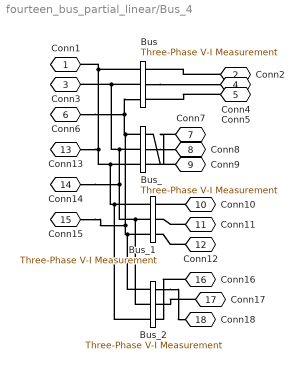
== system fourteen_bus_partial_linear/Bus_4 ==
  Bus : powerlib/Measurements/Three-Phase V-I Measurement  VoltageMeasurement=phase-to-phase  SetLabelV=on  LabelV=VB_4  Vpu=off  VpuLL=off  CurrentMeasurement=yes  SetLabelI=on  LabelI=IB_4  Ipu=off  Pbase=100e6  Vbase=500e3  OutputType=Complex  PhasorSimulation=off  PSBequivalent=0
  Bus_ : powerlib/Measurements/Three-Phase V-I Measurement  VoltageMeasurement=phase-to-phase  SetLabelV=on  LabelV=V_B44  Vpu=off  VpuLL=off  CurrentMeasurement=yes  SetLabelI=on  LabelI=I_B44  Ipu=off  Pbase=100e6  Vbase=500e3  OutputType=Complex  PhasorSimulation=off  PSBequivalent=0
  Bus_1 : powerlib/Measurements/Three-Phase V-I Measurement  VoltageMeasurement=phase-to-phase  SetLabelV=on  LabelV=V_B4  Vpu=off  VpuLL=off  CurrentMeasurement=yes  SetLabelI=on  LabelI=I_B4  Ipu=off  Pbase=100e6  Vbase=500e3  OutputType=Complex  PhasorSimulation=off  PSBequivalent=0
  Bus_2 : powerlib/Measurements/Three-Phase V-I Measurement  VoltageMeasurement=phase-to-phase  SetLabelV=on  LabelV=V_B4_4  Vpu=off  VpuLL=off  CurrentMeasurement=yes  SetLabelI=on  LabelI=I_B4_4  Ipu=off  Pbase=100e6  Vbase=500e3  OutputType=Complex  PhasorSimulation=off  PSBequivalent=0
  Conn1 : PMIOPort  Side=Left
  Conn2 : PMIOPort  Port=2  Side=Right
  Conn3 : PMIOPort  Port=3  Side=Left
  Conn4 : PMIOPort  Port=4  Side=Right
  Conn5 : PMIOPort  Port=5  Side=Right
  Conn6 : PMIOPort  Port=6  Side=Left
  Conn7 : PMIOPort  Port=7  Side=Right
  Conn8 : PMIOPort  Port=8  Side=Right
  Conn9 : PMIOPort  Port=9  Side=Right
  Conn10 : PMIOPort  Port=10  Side=Right
  Conn11 : PMIOPort  Port=11  Side=Right
  Conn12 : PMIOPort  Port=12  Side=Right
  Conn13 : PMIOPort  Port=13  Side=Left
  Conn14 : PMIOPort  Port=14  Side=Left
  Conn15 : PMIOPort  Port=15  Side=Left
  Conn16 : PMIOPort  Port=16  Side=Right
  Conn17 : PMIOPort  Port=17  Side=Right
  Conn18 : PMIOPort  Port=18  Side=Right
  connections:
  Bus/LConn1 -- Conn1/RConn1 -- Bus_2/LConn3 -- Bus_1/LConn1 -- Bus_/LConn3 -- Conn13/RConn1
  Conn3/RConn1 -- Bus/LConn2 -- Bus_/LConn2 -- Bus_2/LConn2 -- Bus_1/LConn2 -- Conn14/RConn1
  Bus_/RConn2 -- Conn8/RConn1
  Bus/RConn2 -- Conn4/RConn1
  Bus/LConn3 -- Conn6/RConn1 -- Bus_/LConn1 -- Bus_2/LConn1 -- Bus_1/LConn3 -- Conn15/RConn1
  Conn10/RConn1 -- Bus_1/RConn1
  Conn11/RConn1 -- Bus_1/RConn2
  Conn12/RConn1 -- Bus_1/RConn3
  Conn9/RConn1 -- Bus_/RConn1
  Conn7/RConn1 -- Bus_/RConn3
  Conn5/RConn1 -- Bus/RConn3
  Conn2/RConn1 -- Bus/RConn1
  Conn17/RConn1 -- Bus_2/RConn2
  Conn16/RConn1 -- Bus_2/RConn3
  Bus_2/RConn1 -- Conn18/RConn1

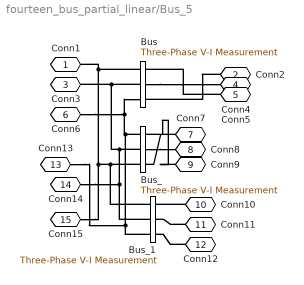
== system fourteen_bus_partial_linear/Bus_5 ==
  Bus : powerlib/Measurements/Three-Phase V-I Measurement  VoltageMeasurement=phase-to-phase  SetLabelV=on  LabelV=VB_5  Vpu=off  VpuLL=off  CurrentMeasurement=yes  SetLabelI=on  LabelI=IB_5  Ipu=off  Pbase=100e6  Vbase=500e3  OutputType=Complex  PhasorSimulation=off  PSBequivalent=0
  Bus_ : powerlib/Measurements/Three-Phase V-I Measurement  VoltageMeasurement=phase-to-phase  SetLabelV=on  LabelV=V_B55  Vpu=off  VpuLL=off  CurrentMeasurement=yes  SetLabelI=on  LabelI=I_B55  Ipu=off  Pbase=100e6  Vbase=500e3  OutputType=Complex  PhasorSimulation=off  PSBequivalent=0
  Bus_1 : powerlib/Measurements/Three-Phase V-I Measurement  VoltageMeasurement=phase-to-phase  SetLabelV=on  LabelV=V_B5  Vpu=off  VpuLL=off  CurrentMeasurement=yes  SetLabelI=on  LabelI=I_B5  Ipu=off  Pbase=100e6  Vbase=500e3  OutputType=Complex  PhasorSimulation=off  PSBequivalent=0
  Conn1 : PMIOPort  Side=Left
  Conn2 : PMIOPort  Port=2  Side=Right
  Conn3 : PMIOPort  Port=3  Side=Left
  Conn4 : PMIOPort  Port=4  Side=Right
  Conn5 : PMIOPort  Port=5  Side=Right
  Conn6 : PMIOPort  Port=6  Side=Left
  Conn7 : PMIOPort  Port=7  Side=Right
  Conn8 : PMIOPort  Port=8  Side=Right
  Conn9 : PMIOPort  Port=9  Side=Right
  Conn10 : PMIOPort  Port=10  Side=Right
  Conn11 : PMIOPort  Port=11  Side=Right
  Conn12 : PMIOPort  Port=12  Side=Right
  Conn13 : PMIOPort  Port=13  Side=Left
  Conn14 : PMIOPort  Port=14  Side=Left
  Conn15 : PMIOPort  Port=15  Side=Left
  connections:
  Conn12/RConn1 -- Bus_1/RConn3
  Conn11/RConn1 -- Bus_1/RConn2
  Conn10/RConn1 -- Bus_1/RConn1
  Bus_1/LConn3 -- Conn13/RConn1 -- Bus_/LConn1 -- Conn6/RConn1 -- Bus/LConn3
  Bus/RConn2 -- Conn4/RConn1
  Bus_/RConn2 -- Conn8/RConn1
  Conn14/RConn1 -- Bus_1/LConn2 -- Bus_/LConn2 -- Bus/LConn2 -- Conn3/RConn1
  Bus_/LConn3 -- Bus_1/LConn1 -- Conn1/RConn1 -- Bus/LConn1 -- Conn15/RConn1
  Conn7/RConn1 -- Bus_/RConn3
  Conn9/RConn1 -- Bus_/RConn1
  Conn5/RConn1 -- Bus/RConn1
  Conn2/RConn1 -- Bus/RConn3

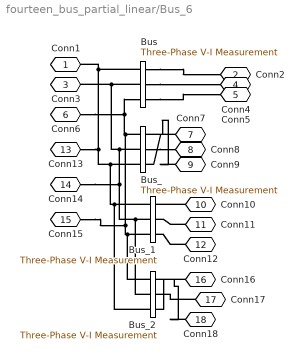
== system fourteen_bus_partial_linear/Bus_6 ==
  Bus : powerlib/Measurements/Three-Phase V-I Measurement  VoltageMeasurement=phase-to-phase  SetLabelV=on  LabelV=VB_6  Vpu=off  VpuLL=off  CurrentMeasurement=yes  SetLabelI=on  LabelI=IB_6  Ipu=off  Pbase=100e6  Vbase=500e3  OutputType=Complex  PhasorSimulation=off  PSBequivalent=0
  Bus_ : powerlib/Measurements/Three-Phase V-I Measurement  VoltageMeasurement=phase-to-phase  SetLabelV=on  LabelV=V_B66  Vpu=off  VpuLL=off  CurrentMeasurement=yes  SetLabelI=on  LabelI=I_B66  Ipu=off  Pbase=100e6  Vbase=500e3  OutputType=Complex  PhasorSimulation=off  PSBequivalent=0
  Bus_1 : powerlib/Measurements/Three-Phase V-I Measurement  VoltageMeasurement=phase-to-phase  SetLabelV=on  LabelV=V_B6  Vpu=off  VpuLL=off  CurrentMeasurement=yes  SetLabelI=on  LabelI=I_B6  Ipu=off  Pbase=100e6  Vbase=500e3  OutputType=Complex  PhasorSimulation=off  PSBequivalent=0
  Bus_2 : powerlib/Measurements/Three-Phase V-I Measurement  VoltageMeasurement=phase-to-phase  SetLabelV=on  LabelV=V_B6_6  Vpu=off  VpuLL=off  CurrentMeasurement=yes  SetLabelI=on  LabelI=I_B6_6  Ipu=off  Pbase=100e6  Vbase=500e3  OutputType=Complex  PhasorSimulation=off  PSBequivalent=0
  Conn1 : PMIOPort  Side=Left
  Conn2 : PMIOPort  Port=2  Side=Right
  Conn3 : PMIOPort  Port=3  Side=Left
  Conn4 : PMIOPort  Port=4  Side=Right
  Conn5 : PMIOPort  Port=5  Side=Right
  Conn6 : PMIOPort  Port=6  Side=Left
  Conn7 : PMIOPort  Port=7  Side=Right
  Conn8 : PMIOPort  Port=8  Side=Right
  Conn9 : PMIOPort  Port=9  Side=Right
  Conn10 : PMIOPort  Port=10  Side=Right
  Conn11 : PMIOPort  Port=11  Side=Right
  Conn12 : PMIOPort  Port=12  Side=Right
  Conn13 : PMIOPort  Port=13  Side=Left
  Conn14 : PMIOPort  Port=14  Side=Left
  Conn15 : PMIOPort  Port=15  Side=Left
  Conn16 : PMIOPort  Port=16  Side=Right
  Conn17 : PMIOPort  Port=17  Side=Right
  Conn18 : PMIOPort  Port=18  Side=Right
  connections:
  Conn17/RConn1 -- Bus_2/RConn2
  Conn12/RConn1 -- Bus_1/RConn3
  Conn11/RConn1 -- Bus_1/RConn2
  Conn10/RConn1 -- Bus_1/RConn1
  Bus/RConn3 -- Conn5/RConn1
  Bus/RConn1 -- Conn2/RConn1
  Bus_2/LConn1 -- Bus_1/LConn3 -- Conn15/RConn1 -- Bus_/LConn1 -- Conn6/RConn1 -- Bus/LConn3
  Bus/RConn2 -- Conn4/RConn1
  Bus_/RConn2 -- Conn8/RConn1
  Bus_2/LConn2 -- Bus_1/LConn2 -- Conn14/RConn1 -- Bus_/LConn2 -- Bus/LConn2 -- Conn3/RConn1
  Bus_2/LConn3 -- Bus_1/LConn1 -- Bus_/LConn3 -- Conn13/RConn1 -- Conn1/RConn1 -- Bus/LConn1
  Conn7/RConn1 -- Bus_/RConn3
  Conn9/RConn1 -- Bus_/RConn1
  Conn16/RConn1 -- Bus_2/RConn3
  Conn18/RConn1 -- Bus_2/RConn1

== system fourteen_bus_partial_linear/Bus_7 ==
  Bus : powerlib/Measurements/Three-Phase V-I Measurement  VoltageMeasurement=phase-to-phase  SetLabelV=on  LabelV=VB_7  Vpu=off  VpuLL=off  CurrentMeasurement=yes  SetLabelI=on  LabelI=IB_7  Ipu=off  Pbase=100e6  Vbase=500e3  OutputType=Complex  PhasorSimulation=off  PSBequivalent=0
  Bus_ : powerlib/Measurements/Three-Phase V-I Measurement  VoltageMeasurement=phase-to-phase  SetLabelV=on  LabelV=V_B7  Vpu=off  VpuLL=off  CurrentMeasurement=yes  SetLabelI=on  LabelI=I_B7  Ipu=off  Pbase=100e6  Vbase=500e3  OutputType=Complex  PhasorSimulation=off  PSBequivalent=0
  Conn1 : PMIOPort  Side=Left
  Conn2 : PMIOPort  Port=2  Side=Right
  Conn3 : PMIOPort  Port=3  Side=Left
  Conn4 : PMIOPort  Port=4  Side=Right
  Conn5 : PMIOPort  Port=5  Side=Right
  Conn6 : PMIOPort  Port=6  Side=Left
  Conn7 : PMIOPort  Port=7  Side=Right
  Conn8 : PMIOPort  Port=8  Side=Right
  Conn9 : PMIOPort  Port=9  Side=Right
  connections:
  Bus_/LConn3 -- Bus/LConn1 -- Conn6/RConn1
  Conn3/RConn1 -- Bus_/LConn2 -- Bus/LConn2
  Bus_/RConn2 -- Conn8/RConn1
  Bus/RConn2 -- Conn4/RConn1
  Bus_/LConn1 -- Conn1/RConn1 -- Bus/LConn3
  Bus_/RConn1 -- Conn7/RConn1
  Bus_/RConn3 -- Conn9/RConn1
  Conn2/RConn1 -- Bus/RConn3
  Conn5/RConn1 -- Bus/RConn1
